simulink library "hcu_lib"  (R2021b)
settings: Solver=VariableStepAuto  StartTime=0.0  StopTime=10.0  RelTol=1e-3
undefined symbols (not defined in the file): ENUM_FAULTSTATE_FAIL, ENUM_FAULTSTATE_INDETERMINATE, ENUM_FAULTSTATE_PASS, EPSILON, FALSE, KPH2MPH, KPH2MPS, KXX2XX, MPH2KPH, MPS2KPH, ONE_INT, ONE_INT16, ONE_INT32, RADPS2RPM, RPM2RADPS, slcm, TRUE, UNDEFINED_VALUE, XX2KXX, ZERO_FLOAT, ZERO_INT, ZERO_INT16, ZERO_INT32
libraries: $bdroot x29, simulink x12, afl x1
(part 3 of 3)

== system hcu_lib/IO_Signal_Process_Blocks/digital_signal_process/fault_filter_reset ==
  i_deb : Inport
  sat : Inport  Port=2
  inc : Inport  Port=3
  dec : Inport  Port=4
  Add : Sum
  Add1 : Sum  Inputs=+-
  Constant : Constant  Value=0  OutDataTypeStr=uint8
  Data Type Conversion : DataTypeConversion  OutDataTypeStr=int16
  MinMax : MinMax  Function=max  Inputs=2
  MinMax1 : MinMax  Inputs=2
  Relational Operator : RelationalOperator  OutDataTypeStr=boolean  RndMeth=Nearest
  Switch : Switch  Criteria=u2 ~= 0
  Unit Delay : UnitDelay  SampleTime=-1  HasFrameUpgradeWarning=on
  fault_flg : Outport
  ff_count : Outport  Port=2
  wires:
  Data Type Conversion/1 -> MinMax/1
  Switch/1 -> Data Type Conversion/1
  Add1/1 -> Switch/3
  Add/1 -> Switch/1
  Relational Operator/1 -> fault_flg/1
  sat/1 -> Relational Operator/2, MinMax1/2  "sat"
  MinMax1/1 -> Relational Operator/1, Unit Delay/1, ff_count/1
  MinMax/1 -> MinMax1/1
  Constant/1 -> MinMax/2
  Unit Delay/1 -> Add1/1, Add/1
  i_deb/1 -> Switch/2  "i_deb"
  dec/1 -> Add1/2  "dec"
  inc/1 -> Add/2  "inc"

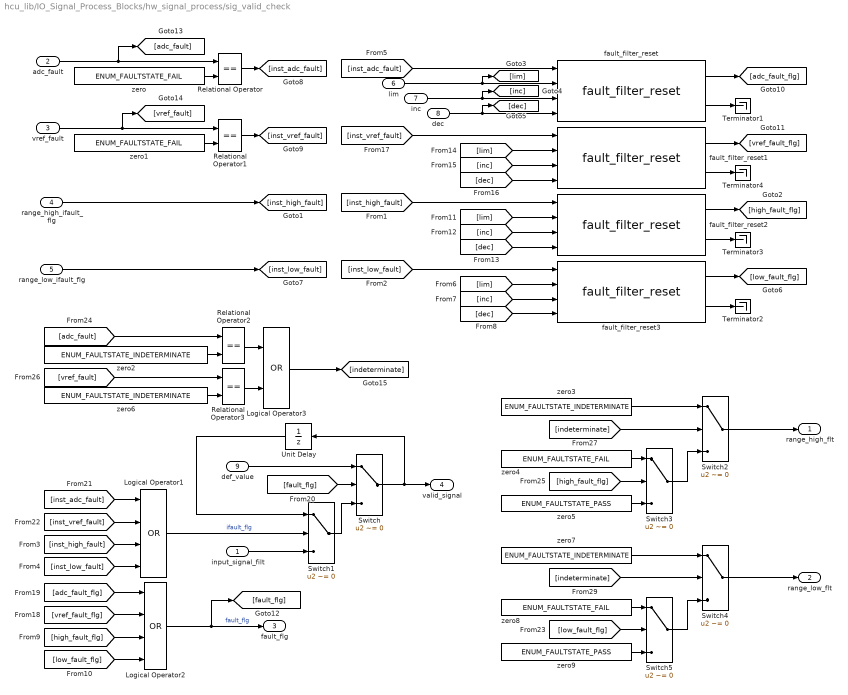
== system hcu_lib/IO_Signal_Process_Blocks/hw_signal_process/sig_valid_check ==
  input_signal_filt : Inport
  adc_fault : Inport  Port=2
  vref_fault : Inport  Port=3
  range_high_ifault_flg : Inport  Port=4
  range_low_ifault_flg : Inport  Port=5
  lim : Inport  Port=6
  inc : Inport  Port=7
  dec : Inport  Port=8
  def_value : Inport  Port=9
  Logical Operator1 : Logic  Operator=OR  Inputs=4  AllPortsSameDT=off  OutDataTypeStr=boolean
  Logical Operator2 : Logic  Operator=OR  Inputs=4  AllPortsSameDT=off  OutDataTypeStr=boolean
  Logical Operator3 : Logic  Operator=OR  AllPortsSameDT=off  OutDataTypeStr=boolean
  Relational Operator{,1..3} (4 alike) : RelationalOperator  Operator===  OutDataTypeStr=boolean  RndMeth=Nearest
  Switch{,1..5} (6 alike) : Switch  Criteria=u2 ~= 0
  Terminator{1..4} (4 alike) : Terminator
  Unit Delay : UnitDelay  SampleTime=-1  HasFrameUpgradeWarning=on
  fault_filter_reset{,1..3} (4 alike) : $bdroot/Signal_Process_Blocks/fault_filter_reset
  zero{,1,4,8} (4 alike) : Constant  Tag=struct('comment',struct('text','','placement',1),'output',struct('width',1,'name','$S_$B','unit','','type','Int16','offset',0,'max',NaN,'min',NaN,'freeze',1,'lsb',1,'arb',0,'class','default','address','','description','','value','0','tolerance',1,'show',0),'date',731455.58675544)  Value=ENUM_FAULTSTATE_FAIL
  zero{2..3,6..7} (4 alike) : Constant  Tag=struct('comment',struct('text','','placement',1),'output',struct('width',1,'name','$S_$B','unit','','type','Int16','offset',0,'max',NaN,'min',NaN,'freeze',1,'lsb',1,'arb',0,'class','default','address','','description','','value','0','tolerance',1,'show',0),'date',731455.58675544)  Value=ENUM_FAULTSTATE_INDETERMINATE
  zero5 : Constant  Tag=struct('comment',struct('text','','placement',1),'output',struct('width',1,'name','$S_$B','unit','','type','Int16','offset',0,'max',NaN,'min',NaN,'freeze',1,'lsb',1,'arb',0,'class','default','address','','description','','value','0','tolerance',1,'show',0),'date',731455.58675544)  Value=ENUM_FAULTSTATE_PASS
  zero9 : Constant  Tag=struct('comment',struct('text','','placement',1),'output',struct('width',1,'name','$S_$B','unit','','type','Int16','offset',0,'max',NaN,'min',NaN,'freeze',1,'lsb',1,'arb',0,'class','default','address','','description','','value','0','tolerance',1,'show',0),'date',731455.58675544)  Value=ENUM_FAULTSTATE_PASS
  range_high_flt : Outport
  range_low_flt : Outport  Port=2
  fault_flg : Outport  Port=3
  valid_signal : Outport  Port=4
  wires:
  Unit Delay/1 -> Switch1/1
  [fault_flg] -> Switch/2
  [inst_low_fault] -> fault_filter_reset3/1
  Switch/1 -> Unit Delay/1, valid_signal/1
  Switch1/1 -> Switch/3
  def_value/1 -> Switch/1
  dec/1 -> [dec], fault_filter_reset/4
  inc/1 -> [inc], fault_filter_reset/3
  lim/1 -> [lim], fault_filter_reset/2
  range_high_ifault_flg/1 -> [inst_high_fault]
  input_signal_filt/1 -> Switch1/3
  Logical Operator1/1 -> Switch1/2  "ifault_flg"
  range_low_ifault_flg/1 -> [inst_low_fault]
  fault_filter_reset3/1 -> [low_fault_flg]
  fault_filter_reset/2 -> Terminator1/1
  fault_filter_reset3/2 -> Terminator2/1
  [lim] -> fault_filter_reset3/2
  [inc] -> fault_filter_reset3/3
  [dec] -> fault_filter_reset3/4
  adc_fault/1 -> Relational Operator/1, [adc_fault]
  zero/1 -> Relational Operator/2
  zero1/1 -> Relational Operator1/2
  vref_fault/1 -> Relational Operator1/1, [vref_fault]
  Relational Operator/1 -> [inst_adc_fault]
  Relational Operator1/1 -> [inst_vref_fault]
  [lim] -> fault_filter_reset2/2
  [inc] -> fault_filter_reset2/3
  [dec] -> fault_filter_reset2/4
  [inst_vref_fault] -> fault_filter_reset1/1
  [lim] -> fault_filter_reset1/2
  [inc] -> fault_filter_reset1/3
  [dec] -> fault_filter_reset1/4
  fault_filter_reset2/2 -> Terminator3/1
  fault_filter_reset1/2 -> Terminator4/1
  fault_filter_reset1/1 -> [vref_fault_flg]
  [inst_adc_fault] -> fault_filter_reset/1
  fault_filter_reset/1 -> [adc_fault_flg]
  [inst_high_fault] -> fault_filter_reset2/1
  fault_filter_reset2/1 -> [high_fault_flg]
  [adc_fault_flg] -> Logical Operator2/1
  [vref_fault_flg] -> Logical Operator2/2
  [high_fault_flg] -> Logical Operator2/3
  [low_fault_flg] -> Logical Operator2/4
  Logical Operator2/1 -> fault_flg/1, [fault_flg]  "fault_flg"
  [inst_adc_fault] -> Logical Operator1/1
  [inst_vref_fault] -> Logical Operator1/2
  [inst_high_fault] -> Logical Operator1/3
  [inst_low_fault] -> Logical Operator1/4
  zero2/1 -> Relational Operator2/2
  [high_fault_flg] -> Switch3/2
  Switch3/1 -> Switch2/3
  zero3/1 -> Switch2/1
  [adc_fault] -> Relational Operator2/1
  zero4/1 -> Switch3/1
  zero5/1 -> Switch3/3
  Switch2/1 -> range_high_flt/1
  zero6/1 -> Relational Operator3/2
  [vref_fault] -> Relational Operator3/1
  Relational Operator2/1 -> Logical Operator3/1
  Relational Operator3/1 -> Logical Operator3/2
  [indeterminate] -> Switch2/2
  Logical Operator3/1 -> [indeterminate]
  [low_fault_flg] -> Switch5/2
  Switch5/1 -> Switch4/3
  zero7/1 -> Switch4/1
  zero8/1 -> Switch5/1
  zero9/1 -> Switch5/3
  [indeterminate] -> Switch4/2
  Switch4/1 -> range_low_flt/1

== system hcu_lib/IO_Signal_Process_Blocks/hw_signal_process/signal_filter ==
  raw_input : Inport
  Tc : Inport  Port=2
  Ts : Inport  Port=3
  FirstOrderFilter : $bdroot/Basic_Blocks/FirstOrderFilter
  IC : UnitDelay  Tag=struct('comment',struct('text','','placement',1),'logdata',struct('maxnumvals',inf,'plotchannels',[],'stepsize',0,'downsampling',1,'loggingmode',3,'channels',1),'output',struct('width',1,'name','$S_$B','unit','','type','Int16','offset',0,'max',NaN,'min',NaN,'freeze',1,'lsb',1,'arb',0,'class','default','address','','description','','autoscalingmode',1,'lowerheadroom',1,'upperheadroom',1,'headroomunit','bit','checkmin',0,'checkmax',0,'show',0,'initial','2'),'state',0,'dt','-1','date',731455.586925799)  SampleTime=-1  HasFrameUpgradeWarning=on
  Switch1 : Switch  Tag=struct('comment',struct('text','','placement',1),'logdata',struct('maxnumvals',inf,'plotchannels',[],'stepsize',0,'downsampling',1,'loggingmode',3,'channels',1),'output',struct('width',1,'name','$S_$B','unit','','type','Int32Bin15','offset',0,'max',65535,'min',-65536,'freeze',1,'lsb',2^-15,'arb',0,'class','default','address','','description','','autoscalingmode',1,'lowerheadroom',1,'upperheadroom',1,'headroomunit','bit','checkmin',0,'checkmax',0,'show',0),'threshold',struct('width',1,'name','$S_$B_threshold','unit','','type','Int16','offset',0,'max',NaN,'min',NaN,'freeze',1,'lsb',1,'arb',0,'class','default','address','','description','','value','1','scalar',0),'date',731455.58657044)  Threshold=0.5  InputSameDT=on
  zero : Constant  Tag=struct('comment',struct('text','','placement',1),'output',struct('width',1,'name','$S_$B','unit','','type','Int16','offset',0,'max',NaN,'min',NaN,'freeze',1,'lsb',1,'arb',0,'class','default','address','','description','','value','0','tolerance',1,'show',0),'date',731455.58675544)  Value=TRUE
  raw_input_filt : Outport
  wires:
  Switch1/1 -> raw_input_filt/1
  FirstOrderFilter/1 -> Switch1/1
  IC/1 -> Switch1/2
  Ts/1 -> FirstOrderFilter/3
  Tc/1 -> FirstOrderFilter/2
  raw_input/1 -> Switch1/3, FirstOrderFilter/1
  zero/1 -> IC/1

== stateflow chart hcu_lib/Basic_Blocks/Minutes_Counter/Scheduler ==
  state trigger_1min
    (default) -> (junction 63) : {
        | counter = 0;
        | }
    trigger_1min -> (junction 63)
    (junction 63) -> (junction 41) [order 1] : [trigger]
    (junction 63) -> (junction 68) [order 2] : {
        | trig_1min = 0;
        | }
    (junction 41) -> (junction 1) : {
        | counter++;
        | }
    (junction 1) -> (junction 8) [order 1] : [counter%%uint32((60*1/task_time_s)) == 0]  /* 1min trigger */
    (junction 1) -> (junction 5) [order 2] : {
        | trig_1min = 0;
        | }
    (junction 8) -> (junction 9) : {
        | trig_1min = 1;
        | counter = 0;
        | }
  data: counter local uint32 size=1; task_time_s input; trigger input; trig_1min output boolean

== stateflow chart hcu_lib/Basic_Blocks/Seconds_Counter/Scheduler ==
  state trigger_1sec
    (default) -> (junction 63) : {
        | counter = 0;
        | }
    trigger_1sec -> (junction 63)
    (junction 63) -> (junction 41) [order 1] : [trigger]
    (junction 63) -> (junction 68) [order 2] : {
        | trig_1sec = 0;
        | }
    (junction 41) -> (junction 1) : {
        | counter++;
        | }
    (junction 1) -> (junction 8) [order 1] : [counter%%uint32(1/task_time_s) == 0]  /* 1sec trigger */
    (junction 1) -> (junction 5) [order 2] : {
        | trig_1sec = 0;
        | }
    (junction 8) -> (junction 9) : {
        | trig_1sec = 1;
        | counter = 0;
        | }
  data: counter local uint32 size=1; task_time_s input; trigger input; trig_1sec output boolean

== stateflow chart hcu_lib/Basic_Blocks/RangeTimer/Scheduler ==
  state trigger_1sec
    (default) -> (junction 63) : {
        | counter = 0;
        | }
    trigger_1sec -> (junction 63)
    (junction 63) -> (junction 41) [order 1] : [trigger]
    (junction 63) -> (junction 68) [order 2] : {
        | trig_1sec = 0;
        | }
    (junction 41) -> (junction 1) : {
        | counter++;
        | }
    (junction 1) -> (junction 8) [order 1] : [counter%%uint32(1/task_time_s) == 0]  /* 1sec trigger */
    (junction 1) -> (junction 5) [order 2] : {
        | trig_1sec = 0;
        | }
    (junction 8) -> (junction 9) : {
        | trig_1sec = 1;
        | counter = 0;
        | }
  data: counter local uint32 size=1; task_time_s input; trigger input; trig_1sec output boolean

== stateflow chart hcu_lib/Signal_Process_Blocks/latching_fault_filter/lff_ctl ==
  (default) -> (junction 9)
  (junction 9) -> (junction 13) [order 1] : [i_fault]
      | {count+=inc;}
  (junction 9) -> (junction 13) [order 2] : {count-=dec;}
  (junction 13) -> (junction 10)
  (junction 10) -> (junction 11) [order 1] : [count>=sat]
      | {count=sat;
      | fault_flg=1;}
  (junction 10) -> (junction 11) [order 2] : [count<=0]
      | {count=0;}
  (junction 10) -> (junction 11) [order 3]
  (junction 11) -> (junction 12) : {ff_count = count;}
  data: sat input uint8; inc input uint8; dec input uint8; i_fault input boolean; fault_flg output boolean =0; ff_count output uint8; count local int16 =0

== stateflow chart hcu_lib/Signal_Process_Blocks/latching fault filter reinit/lff_ctl ==
  (default) -> (junction 25)
  (junction 25) -> (junction 27) [order 1] : [reinit]
  (junction 25) -> (junction 20) [order 2]
  (junction 27) -> (junction 28) : {fault_flg = FALSE;
      |  count = 0;}
  (junction 20) -> (junction 29) [order 1] : [i_fault]
  (junction 20) -> (junction 24) [order 2] : {count-=dec;}
  (junction 29) -> (junction 30) : {count+=inc;}
  (junction 30) -> (junction 24)
  (junction 24) -> (junction 21)
  (junction 21) -> (junction 31) [order 1] : [count >= sat]
  (junction 21) -> (junction 26) [order 2]
  (junction 31) -> (junction 32) : {count = sat;
      | fault_flg = TRUE;}
  (junction 26) -> (junction 34) [order 1] : [count <= 0]
  (junction 26) -> (junction 22) [order 2]
  (junction 34) -> (junction 33) : {count = 0;}
  (junction 33) -> (junction 22)
  (junction 32) -> (junction 33)
  (junction 28) -> (junction 32)
  (junction 22) -> (junction 23) : {ff_count = count;}
  data: sat input uint8; inc input uint8; dec input uint8; i_fault input boolean; fault_flg output boolean =0; ff_count output uint8; count local int16 =0; TRUE parameter boolean; FALSE parameter boolean; reinit input boolean
